simulink model "raspberrypi_motion_sensor_camera"  (R2018b)
settings: Solver=FixedStepDiscrete  StartTime=0.0  StopTime=inf  RelTol=1e-3  EnableMultiTasking=on
libraries: embdlinuxlib x4, realtime_examples_misc x1, simulink x1
settings Model: SimulationMode=external  ExtModeTrigDuration=100  Creator=The MathWorks, Inc.  LastModifiedBy=The MathWorks, Inc.
settings SolverCC: PositivePriorityOrder=on
settings DataIOCC: LimitDataPoints=on  SaveFormat=Array
settings OptimizationCC: ExpressionDepthLimit=2147483647  LifeSpan=Inf  MaxStackSize=64
settings DebuggingCC: UnderspecifiedInitializationDetection=Classic  MergeDetectMultiDrivingBlocksExec=none  AllowSymbolicDim=off  StateNameClashWarn=warning  SFUnexpectedBacktrackingDiag=warning  SFNoUnconditionalDefaultTransitionDiag=warning  SFExecutionAtInitializationDiag=none
settings HardwareCC: ProdBitPerPointer=32  ProdBitPerSizeT=32  ProdBitPerPtrDiffT=32  ProdLargestAtomicInteger=Long  ProdLargestAtomicFloat=Double  ProdWordSize=32  ProdHWDeviceType=ARM Compatible->ARM Cortex  UseEmbeddedCoderFeatures=off  UseSimulinkCoderFeatures=off
settings ModelReferenceCC: PropagateSignalLabelsOutOfModel=off
settings SFSimCC: SimUseLocalCustomCode=off
settings RTWCC: SystemTargetFile=ert.tlc  HardwareBoard=Raspberry Pi  TLCOptions=-aInlineSetEventsForThisBaseRateFcn=TLC_FALSE -aSuppressMultiTaskScheduler=TLC_FALSE -aRateBasedStepFcn=0  TemplateMakefile=ert_default_tmf  GenerateReport=on  RTWVerbose=off  RTWUseLocalCustomCode=off  Toolchain=GNU GCC Raspberry Pi  LaunchReport=on
settings CodeAppCC: ForceParamTrailComments=on  OperatorAnnotations=on  StateflowObjectComments=on  MATLABSourceComments=on
settings ERTTargetCC: MultiwordLength=2048  ERTCustomFileBanners=off  SupportContinuousTime=on  SupportNonInlinedSFcns=on  ModelStepFunctionPrototypeControlCompliant=off
settings ConfigComp: CovMetricSettings=dw  CovHtmlReporting=on  CovSaveCumulativeToWorkspaceVar=on  CovSaveSingleToWorkspaceVar=on  CovShowResultsExplorer=off  CovExternalEMLEnable=off

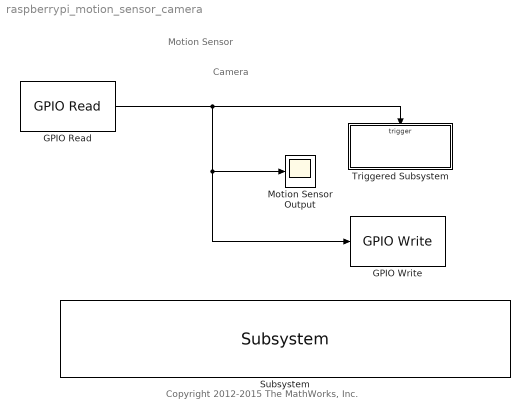
== system raspberrypi_motion_sensor_camera ==
  note: Motion Sensor
  note: Copyright 2012-2015 The MathWorks, Inc.
  note: Camera
  GPIO Read : embdlinuxlib/GPIO Read  board=Model B Rev2  gpio=23  internalResistor=Off  sampleTime=0.1  direction=Input  blockPlatform=Raspberry Pi
      settings: SourceProductName=Simulink Support Package for Raspberry Pi Hardware  SourceProductBaseCode=RASPPI
  GPIO Write : embdlinuxlib/GPIO Write  board=Model B Rev2  gpio=24  direction=Output  blockPlatform=Raspberry Pi
      settings: SourceProductName=Simulink Support Package for Raspberry Pi Hardware  SourceProductBaseCode=RASPPI
  Motion Sensor Output : Scope
  Subsystem : realtime_examples_misc/Subsystem  SystemSampleTime=-1
  Triggered Subsystem : Subsystem  TreatAsAtomicUnit=on
  wires:
  GPIO Read/1 -> GPIO Write/1, Motion Sensor Output/1, Triggered Subsystem/Trigger

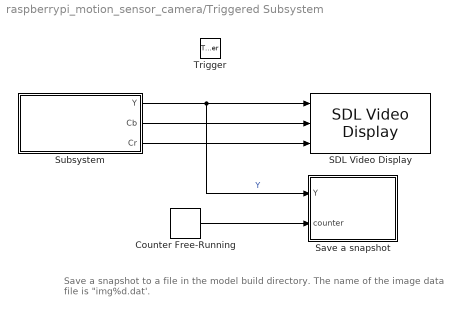
== system raspberrypi_motion_sensor_camera/Triggered Subsystem ==
  note: Save a snapshot to a file in the model build directory. The name
      | of the image data file is "img%d.dat'.
  Trigger : TriggerPort  VariantControl=Variant
  Counter Free-Running : simulink/Sources/Counter Free-Running  NumBits=32  tsamp=-1
  SDL Video Display : embdlinuxlib/SDL Video Display  pixelFormat=YCbCr 4:2:2  pixelOrder=Planar  rowMajor=on  blockPlatform=Raspberry Pi
      settings: SourceProductName=Simulink Support Package for Raspberry Pi Hardware  SourceProductBaseCode=RASPPI
  Save a snapshot : MATLAB Function  TreatAsAtomicUnit=on
  Subsystem : Subsystem
  wires:
  Subsystem/3(Cr) -> SDL Video Display/3
  Subsystem/2(Cb) -> SDL Video Display/2
  Subsystem/1(Y) -> Save a snapshot/1(Y), SDL Video Display/1  "Y"
  Counter Free-Running/1 -> Save a snapshot/2(counter)

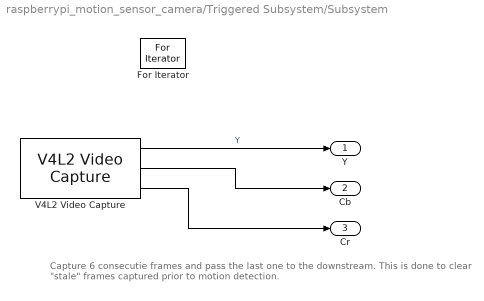
== system raspberrypi_motion_sensor_camera/Triggered Subsystem/Subsystem ==
  note: Capture 6 consecutie frames and pass the last one to the downstream.
      | This is done to clear "stale" frames captured prior to motion detection.
  For Iterator : ForIterator  IterationLimit=6  ShowIterationPort=off
  V4L2 Video Capture : embdlinuxlib/V4L2 Video Capture  m_devName='/dev/video0'  roi=[0, 0, 640, 480]  imSizeSelection=160x120  imSize=[640, 480]  pixelFormat=YCbCr 4:2:2  pixelOrder=Planar  sampleTime=-1  simOutput=Colorbars  blockPlatform=Raspberry Pi
      settings: SourceProductName=Simulink Support Package for Raspberry Pi Hardware  SourceProductBaseCode=RASPPI
  Y : Outport
  Cb : Outport  Port=2
  Cr : Outport  Port=3
  wires:
  V4L2 Video Capture/3 -> Cr/1
  V4L2 Video Capture/1 -> Y/1  "Y"
  V4L2 Video Capture/2 -> Cb/1

== matlab function raspberrypi_motion_sensor_camera/Triggered Subsystem/Save a snapshot ==
  data: Y input; counter input
function fcn(Y, counter)
%#codegen

% Save 160x120 grayscale image to a file
format = ['%d ', 0];
fname  = coder.nullcopy(uint8(zeros(1, 32)));
coder.ceval('sprintf', coder.wref(fname), ['img%d.dat', 0], counter);
fd = coder.opaque('FILE *');
fd = coder.ceval('fopen', fname, ['w', 0]);
for i = 1:160
    for j = 1:120
        coder.ceval('fprintf', fd, format, Y(i, j));
    end
end
coder.ceval('fclose', fd);
